simulink model "FlightGear_Animation"  (R2020a)
settings: Solver=VariableStepAuto  StartTime=0.0  StopTime=100  RelTol=1e-3
undefined symbols (not defined in the file or in its folder): Earth, WGS84
libraries: simulink_extras x3, aerolibtransform2 x1, aerolibfltsims x1, simulink x1
settings Model: Creator=rag  LastModifiedBy=rag
settings SFSimCC: CustomCodeUndefinedFunction=UseInterfaceOnly

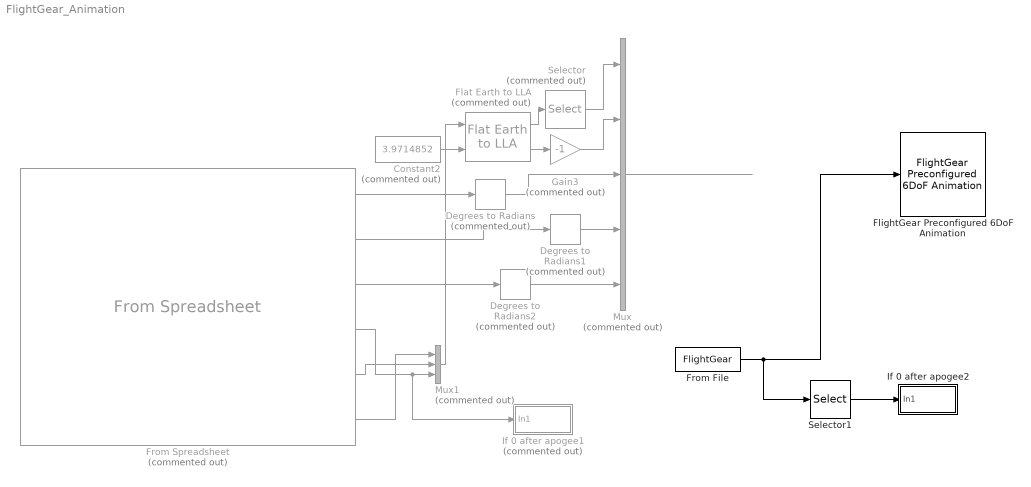
== system FlightGear_Animation ==
  Constant2 : Constant  Commented=on  Value=3.9714852
  Degrees to Radians : simulink_extras/Transformations/Degrees to Radians  Commented=on
  Degrees to Radians1 : simulink_extras/Transformations/Degrees to Radians  Commented=on
  Degrees to Radians2 : simulink_extras/Transformations/Degrees to Radians  Commented=on
  Flat Earth to LLA : aerolibtransform2/Flat Earth to LLA  Commented=on  units=Metric (MKS)  ptype=Earth (WGS84)  F=1/298.257223563  R=6378137  refPosPort=off  LL0=[21.318358277648 -157.9232805920725]  psi=0
  FlightGear Preconfigured 6DoF Animation : aerolibfltsims/FlightGear Preconfigured 6DoF Animation  xFlightGearVersion=v2018.2  DestinationIpAddress=127.0.0.1  DestinationPort=5502  SampleTime=1/50  packetVersion=24
  From File : FromFile  FileName=FlightGear  SampleTime=0  ExtrapolationBeforeFirstDataPoint=Hold first value  ExtrapolationAfterLastDataPoint=Hold last value
  From Spreadsheet : FromSpreadsheet  Commented=on  FileName=C:\Users\rag\Downloads\BPS_Sprint_Flight_8_No_LLA.xlsx  SheetName=BPS_Sprint_Flight_8_No_LLA.xlsx  Range=A1:G1671  ExtrapolationBeforeFirstDataPoint=Hold first value  ExtrapolationAfterLastDataPoint=Hold last value
  Gain3 : Gain  Commented=on  Gain=-1
  If 0 after apogee1 : Subsystem  Commented=on
  If 0 after apogee2 : Subsystem
  Mux : Mux  Commented=on  Inputs=5
  Mux1 : Mux  Commented=on  Inputs=3
  Selector : Selector  Commented=on  InputPortWidth=2  IndexOptions=Index vector (dialog)  Indices=[2 1]  OutputSizes=1
  Selector1 : Selector  InputPortWidth=6  IndexOptions=Index vector (dialog)  Indices=3  OutputSizes=1
  wires:
  Mux/1 -> ?
  From Spreadsheet/1 -> Degrees to Radians/1
  Mux1/1 -> Flat Earth to LLA/1
  Constant2/1 -> Flat Earth to LLA/2
  Flat Earth to LLA/2 -> Gain3/1
  Gain3/1 -> Mux/2
  Selector/1 -> Mux/1
  From Spreadsheet/2 -> Degrees to Radians1/1
  From Spreadsheet/3 -> Degrees to Radians2/1
  From Spreadsheet/6 -> Mux1/1
  Degrees to Radians/1 -> Mux/3
  Degrees to Radians1/1 -> Mux/4
  Degrees to Radians2/1 -> Mux/5
  Flat Earth to LLA/1 -> Selector/1
  From Spreadsheet/5 -> Mux1/2
  From Spreadsheet/4 -> If 0 after apogee1/1(In1), Mux1/3
  From File/1 -> Selector1/1, FlightGear Preconfigured 6DoF Animation/1
  Selector1/1 -> If 0 after apogee2/1(In1)

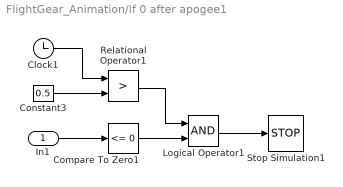
== system FlightGear_Animation/If 0 after apogee1 ==
  In1 : Inport
  Clock1 : Clock
  Compare To Zero1 : simulink/Logic and Bit Operations/Compare To Zero  relop=<=  OutDataTypeStr=boolean
  Constant3 : Constant  Value=0.5
  Logical Operator1 : Logic  AllPortsSameDT=off  OutDataTypeStr=boolean
  Relational Operator1 : RelationalOperator  Operator=>  OutDataTypeStr=boolean  RndMeth=Simplest
  Stop Simulation1 : Stop
  wires:
  Clock1/1 -> Relational Operator1/1
  Constant3/1 -> Relational Operator1/2
  In1/1 -> Compare To Zero1/1
  Logical Operator1/1 -> Stop Simulation1/1
  Compare To Zero1/1 -> Logical Operator1/2
  Relational Operator1/1 -> Logical Operator1/1

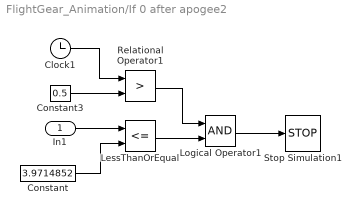
== system FlightGear_Animation/If 0 after apogee2 ==
  In1 : Inport
  Clock1 : Clock
  Constant : Constant  Value=3.9714852
  Constant3 : Constant  Value=0.5
  LessThanOrEqual : RelationalOperator  Operator=<=  OutDataTypeStr=boolean  RndMeth=Simplest
  Logical Operator1 : Logic  AllPortsSameDT=off  OutDataTypeStr=boolean
  Relational Operator1 : RelationalOperator  Operator=>  OutDataTypeStr=boolean  RndMeth=Simplest
  Stop Simulation1 : Stop
  wires:
  Clock1/1 -> Relational Operator1/1
  Constant3/1 -> Relational Operator1/2
  In1/1 -> LessThanOrEqual/1
  Logical Operator1/1 -> Stop Simulation1/1
  LessThanOrEqual/1 -> Logical Operator1/2
  Relational Operator1/1 -> Logical Operator1/1
  Constant/1 -> LessThanOrEqual/2
